simulink model "Time_invariance_Test"  (R2018b)
settings: Solver=VariableStepAuto  StartTime=0.0  StopTime=10.0  RelTol=1e-3
settings Model: Creator=hp  LastModifiedBy=hp

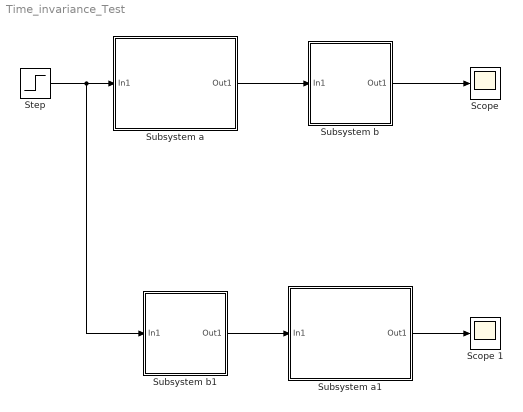
== system Time_invariance_Test ==
  "Scope " : Scope
  Scope 1 : Scope
  "Step " : Step  SampleTime=0
  Subsystem a : Subsystem
  Subsystem a1 : Subsystem
  Subsystem b : Subsystem
  Subsystem b1 : Subsystem
  wires:
  "Step "/1 -> Subsystem b1/1(In1), Subsystem a/1(In1)
  Subsystem a/1(Out1) -> Subsystem b/1(In1)
  Subsystem b/1(Out1) -> "Scope "/1
  Subsystem b1/1(Out1) -> Subsystem a1/1(In1)
  Subsystem a1/1(Out1) -> Scope 1/1

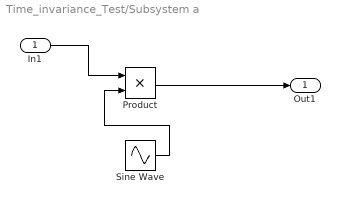
== system Time_invariance_Test/Subsystem a ==
  In1 : Inport
  "Product " : Product
  "Sine Wave " : Sin  SampleTime=0
  Out1 : Outport
  wires:
  "Sine Wave "/1 -> "Product "/2
  In1/1 -> "Product "/1
  "Product "/1 -> Out1/1

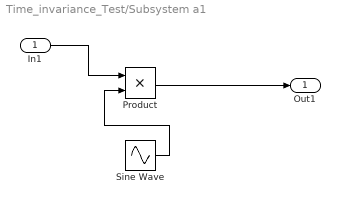
== system Time_invariance_Test/Subsystem a1 ==
  In1 : Inport
  "Product " : Product
  "Sine Wave " : Sin  SampleTime=0
  Out1 : Outport
  wires:
  "Sine Wave "/1 -> "Product "/2
  In1/1 -> "Product "/1
  "Product "/1 -> Out1/1

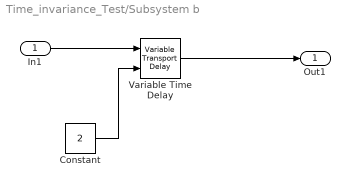
== system Time_invariance_Test/Subsystem b ==
  In1 : Inport
  Constant : Constant  Value=2
  "Variable Time Delay " : VariableTransportDelay  MaximumDelay=10
  Out1 : Outport
  wires:
  "Variable Time Delay "/1 -> Out1/1
  Constant/1 -> "Variable Time Delay "/2
  In1/1 -> "Variable Time Delay "/1

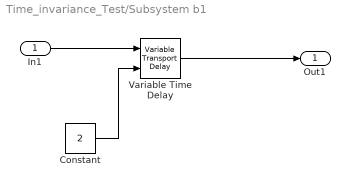
== system Time_invariance_Test/Subsystem b1 ==
  In1 : Inport
  Constant : Constant  Value=2
  "Variable Time Delay " : VariableTransportDelay  MaximumDelay=10
  Out1 : Outport
  wires:
  "Variable Time Delay "/1 -> Out1/1
  Constant/1 -> "Variable Time Delay "/2
  In1/1 -> "Variable Time Delay "/1
